simulink model "weboflies"  (R2020a)
settings: Solver=VariableStepAuto  StartTime=0.0  StopTime=200  RelTol=1e-3
settings Model: Creator=zylee  LastModifiedBy=zylee

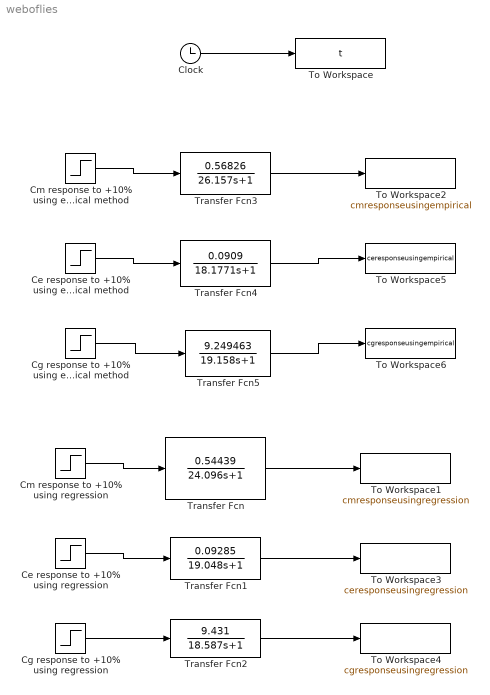
== system weboflies ==
  Ce response to +10% using empirical method : Step  Time=5.8178  Before=1  After=1.1  SampleTime=0
  Ce response to +10% using regression : Step  Time=4.9052  Before=1  After=1.1  SampleTime=0
  Cg response to +10% using empirical method : Step  Time=0  Before=1  After=1.1  SampleTime=0
  Cg response to +10% using regression : Step  Time=0  Before=1  After=1.1  SampleTime=0
  Clock : Clock
  Cm response to +10% using empirical method : Step  Time=8.1512  Before=1  After=1.1  SampleTime=0
  Cm response to +10% using regression : Step  Time=7.8724  Before=1  After=1.1  SampleTime=0
  To Workspace : ToWorkspace  VariableName=t  SampleTime=-1
  To Workspace1 : ToWorkspace  VariableName=cmresponseusingregression  SampleTime=-1
  To Workspace2 : ToWorkspace  VariableName=cmresponseusingempirical  SampleTime=-1
  To Workspace3 : ToWorkspace  VariableName=ceresponseusingregression  SampleTime=-1
  To Workspace4 : ToWorkspace  VariableName=cgresponseusingregression  SampleTime=-1
  To Workspace5 : ToWorkspace  VariableName=ceresponseusingempirical  SampleTime=-1
  To Workspace6 : ToWorkspace  VariableName=cgresponseusingempirical  SampleTime=-1
  Transfer Fcn : TransferFcn  Numerator=[0.54439]  Denominator=[24.096 1]
  Transfer Fcn1 : TransferFcn  Numerator=[0.09285]  Denominator=[19.048 1]
  Transfer Fcn2 : TransferFcn  Numerator=[9.431]  Denominator=[18.587 1]
  Transfer Fcn3 : TransferFcn  Numerator=[0.56826]  Denominator=[26.157 1]
  Transfer Fcn4 : TransferFcn  Numerator=[0.0909]  Denominator=[18.1771 1]
  Transfer Fcn5 : TransferFcn  Numerator=[9.249463]  Denominator=[19.158 1]
  wires:
  Clock/1 -> To Workspace/1
  Cm response to +10% using empirical method/1 -> Transfer Fcn3/1
  Cg response to +10% using regression/1 -> Transfer Fcn2/1
  Ce response to +10% using regression/1 -> Transfer Fcn1/1
  Cm response to +10% using regression/1 -> Transfer Fcn/1
  Ce response to +10% using empirical method/1 -> Transfer Fcn4/1
  Cg response to +10% using empirical method/1 -> Transfer Fcn5/1
  Transfer Fcn/1 -> To Workspace1/1
  Transfer Fcn3/1 -> To Workspace2/1
  Transfer Fcn1/1 -> To Workspace3/1
  Transfer Fcn2/1 -> To Workspace4/1
  Transfer Fcn4/1 -> To Workspace5/1
  Transfer Fcn5/1 -> To Workspace6/1
